simulink library "wheelLibrary"  (R2022b)
settings: Solver=VariableStepAuto  StartTime=0.0  StopTime=10.0  RelTol=1e-3
undefined symbols (not defined in the file): wheel
settings Model: Creator=ericb  LastModifiedBy=ericb
settings SolverCC: AlgebraicLoopSolver=TrustRegion
settings DebuggingCC: UnconnectedInputMsg=warning  UnconnectedOutputMsg=warning  UnconnectedLineMsg=warning  SFMachineParentedDataDiag=warning
settings ModelReferenceCC: EnableRefExpFcnMdlSchedulingChecks=on
settings RTWCC: DLArmComputeVersion=19.05

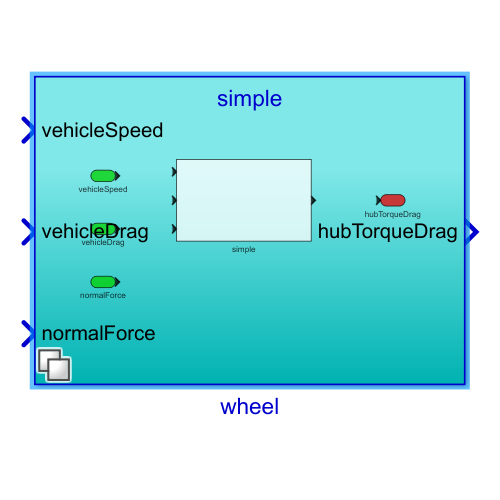
[thumbnail: Simulink's stored preview of the top-level diagram]
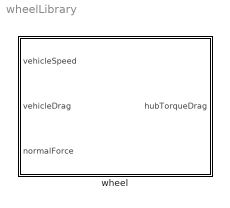
== system wheelLibrary ==
  wheel : Subsystem  Variant=on

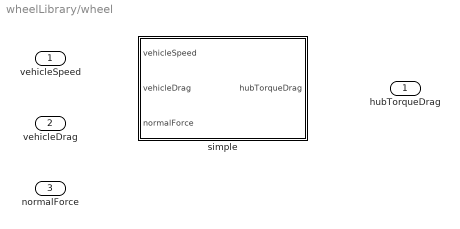
== system wheelLibrary/wheel ==
  vehicleSpeed : Inport
  vehicleDrag : Inport  Port=2
  normalForce : Inport  Port=3
  simple : Subsystem  VariantControl=strcmp(wheel.blockChoice, 'simple')
  hubTorqueDrag : Outport

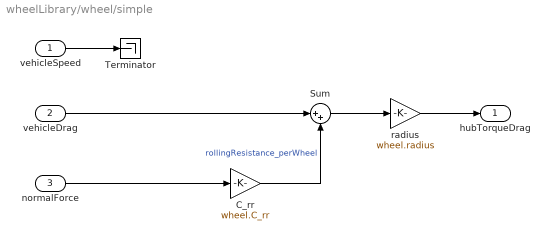
== system wheelLibrary/wheel/simple ==
  vehicleSpeed : Inport
  vehicleDrag : Inport  Port=2
  normalForce : Inport  Port=3
  C_rr : Gain  Gain=wheel.C_rr
  Sum : Sum  Inputs=|++
  Terminator : Terminator
  radius : Gain  Gain=wheel.radius
  hubTorqueDrag : Outport
  wires:
  vehicleSpeed/1 -> Terminator/1
  normalForce/1 -> C_rr/1
  vehicleDrag/1 -> Sum/1
  C_rr/1 -> Sum/2  "rollingResistance_perWheel"
  Sum/1 -> radius/1
  radius/1 -> hubTorqueDrag/1
